simulink model "Q3_a"  (R2017b)
settings: Solver=VariableStepAuto  StartTime=0.0  StopTime=1  RelTol=1e-8  AbsTol=1e-8
undefined symbols (not defined in the file or in its folder): K2
libraries: cstblocks x6
settings Model: Creator=User  LastModifiedBy=User

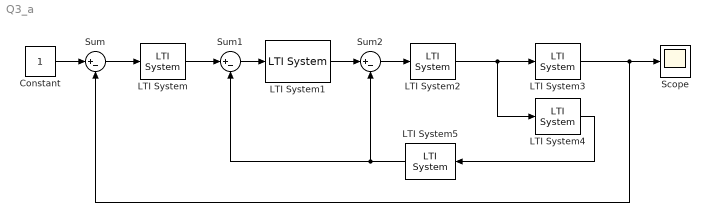
== system Q3_a ==
  Constant : Constant
  LTI System : cstblocks/LTI System  sys=K3  IC=[]
  LTI System1 : cstblocks/LTI System  sys=K2*tf(1,[1 0])  IC=[]
  LTI System2 : cstblocks/LTI System  sys=K1  IC=[]
  LTI System3 : cstblocks/LTI System  sys=Pa  IC=[]
  LTI System4 : cstblocks/LTI System  sys=Pq  IC=[]
  LTI System5 : cstblocks/LTI System  sys=H  IC=[]
  Scope : Scope
  Sum : Sum  Inputs=|+-
  Sum1 : Sum  Inputs=|+-
  Sum2 : Sum  Inputs=|+-
  wires:
  Sum/1 -> LTI System/1
  Constant/1 -> Sum/1
  LTI System/1 -> Sum1/1
  Sum1/1 -> LTI System1/1
  LTI System1/1 -> Sum2/1
  Sum2/1 -> LTI System2/1
  LTI System2/1 -> LTI System4/1, LTI System3/1
  LTI System4/1 -> LTI System5/1
  LTI System5/1 -> Sum1/2, Sum2/2
  LTI System3/1 -> Sum/2, Scope/1
